simulink model "wave_forces"  (R2023a)
settings: Solver=ode4  StartTime=0.0  StopTime=10.0  FixedStep=0.01  RelTol=1e-3
values from neighbouring files (symbols this model uses):
  wave_force_stddev = [0,0,0,0,0,0]    [init_wave_forces.m]
settings Model: Creator=tobiasvt  LastModifiedBy=HalvorPlatou
settings SolverCC: AlgebraicLoopSolver=TrustRegion
settings DebuggingCC: UnconnectedInputMsg=warning  UnconnectedOutputMsg=warning  UnconnectedLineMsg=warning
settings ModelReferenceCC: EnableRefExpFcnMdlSchedulingChecks=on
settings SFSimCC: CustomCodeUndefinedFunction=UseInterfaceOnly
settings RTWCC: Description=FMU based on GRT (Functional Mock-up Unit)  SystemTargetFile=grtfmi.tlc  GenerateMakefile=off  TemplateMakefile=none  RetainRTWFile=on
settings STFCustomTargetCC: ConcurrentExecutionCompliant=off  CombineOutputUpdateFcns=on  CodeInterfacePackaging=Reusable function  GRTInterface=off  GenerateAllocFcn=on  UseToolchainInfoCompliant=off  SystemTargetFile=grtfmi.tlc
settings GRTTargetCC: ParMdlRefBuildCompliant=off  CompOptLevelCompliant=off  ConcurrentExecutionCompliant=off  MatFileLogging=off  CodeInterfacePackaging=Reusable function  CPPClassGenCompliant=off  GenerateAllocFcn=on  UseToolchainInfoCompliant=off

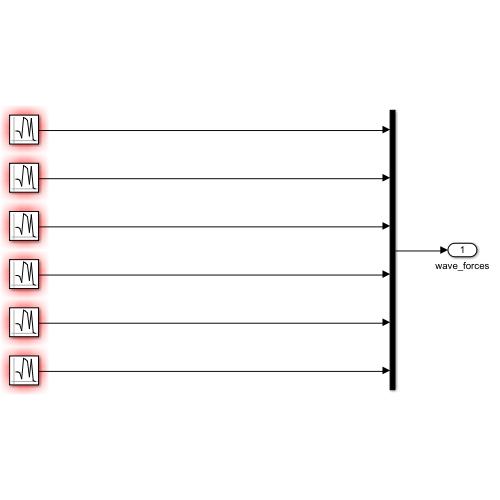
[thumbnail: Simulink's stored preview of the top-level diagram]
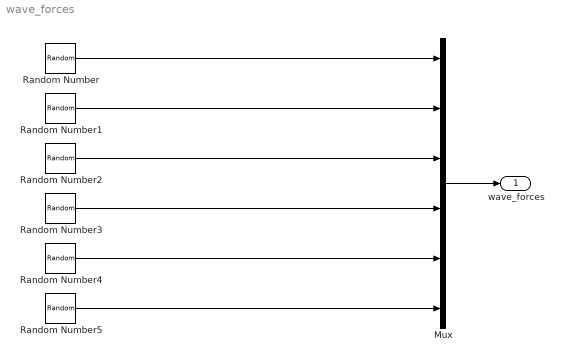
== system wave_forces ==
  Mux : Mux  Inputs=6
  Random Number : RandomNumber  Variance=wave_force_stddev(1)*wave_force_stddev(1)  Seed=111  SampleTime=0.1
  Random Number1 : RandomNumber  Variance=wave_force_stddev(2)*wave_force_stddev(2)  Seed=222  SampleTime=0.1
  Random Number2 : RandomNumber  Variance=wave_force_stddev(3)*wave_force_stddev(3)  Seed=333  SampleTime=0.1
  Random Number3 : RandomNumber  Variance=wave_force_stddev(4)*wave_force_stddev(4)  Seed=444  SampleTime=0.1
  Random Number4 : RandomNumber  Variance=wave_force_stddev(5)*wave_force_stddev(5)  Seed=555  SampleTime=0.1
  Random Number5 : RandomNumber  Variance=wave_force_stddev(6)*wave_force_stddev(6)  Seed=666  SampleTime=0.1
  wave_forces : Outport  VectorParamsAs1DForOutWhenUnconnected=off
  wires:
  Random Number5/1 -> Mux/6
  Random Number/1 -> Mux/1
  Mux/1 -> wave_forces/1
  Random Number4/1 -> Mux/5
  Random Number1/1 -> Mux/2
  Random Number3/1 -> Mux/4
  Random Number2/1 -> Mux/3
